simulink model "linearMSBR"  (R2016b)
settings: Solver=ode45  StartTime=0.0  StopTime=100.0  RelTol=1e-3
values from neighbouring files (symbols this model uses):
  A = zeros(16,16)    [simulinkmatrixconstructor.m]
  B = zeros(16,11)    [simulinkmatrixconstructor.m]
  mdotf_0 = (fPg1+fPg2+fPf1+fPf2+fPf3+fPf3)*P/cpf/(Tfhigh-Tflow)    (= 3034.32428551)    [simulinkmatrixconstructor.m]
  mfuelloop = 25*rhof*(1.32+1.22)    (= 8064.5)    [simulinkmatrixconstructor.m]
libraries: simulink x1
settings Model: Creator=gavin  LastModifiedBy=gavin

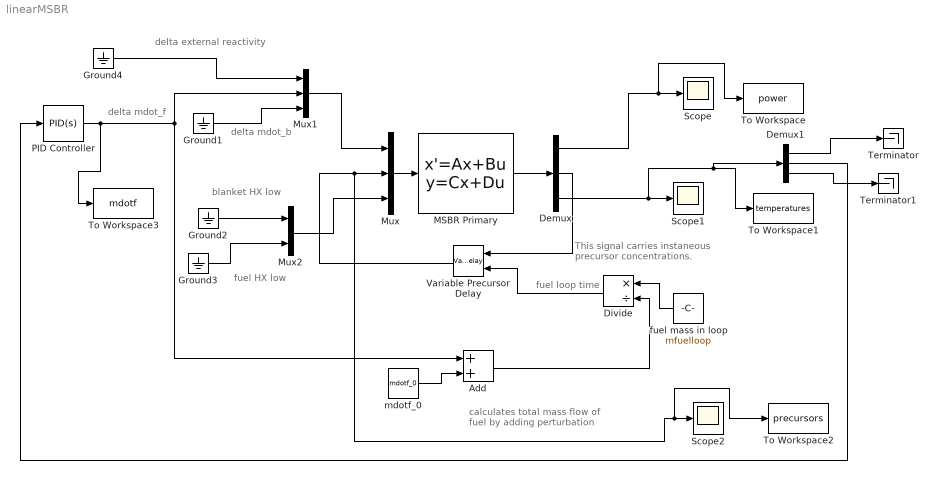
== system linearMSBR ==
  note: fuel HX low
  note: blanket HX low
  note: fuel loop time
  note: calculates total mass flow
      | of fuel by adding perturbation
  note: delta mdot_b
  note: delta mdot_f
  note: delta external reactivity
  note: This signal carries instaneous
      |  precursor concentrations.
  Add : Sum
  Demux : Demux  Outputs=[1 6 9]
  Demux1 : Demux  Outputs=[5 1 3]
  Divide : Product  Inputs=*/
  Ground{1..4} (4 alike) : Ground
  MSBR Primary : StateSpace  A=A  B=B  C=eye(16,16)  D=zeros(16,11)  X0=0  ContinuousStateAttributes='MSBR.state.variables'
  Mux : Mux  Inputs=[3 6 2]
  Mux1 : Mux  Inputs=3
  Mux2 : Mux  Inputs=2
  PID Controller : simulink/Continuous/PID Controller  Controller=PID  TimeDomain=Continuous-time  SampleTime=-1  IntegratorMethod=Forward Euler  FilterMethod=Forward Euler  Form=Parallel  UseFilter=on  ControllerParametersSource=internal  P=200  I=40  D=10  N=0.012270941775282  InitialConditionSource=internal  InitialConditionForIntegrator=0  InitialConditionForFilter=0  ExternalReset=none  LimitOutput=off  UpperSaturationLimit=inf  LowerSaturationLimit=-inf  LinearizeAsGain=on  AntiWindupMode=none  Kb=1  TrackingMode=off  Kt=1  PParamMin=[]  PParamMax=[]  IParamMin=[]  IParamMax=[]  DParamMin=[]  DParamMax=[]  NParamMin=[]  NParamMax=[]  KbParamMin=[]  KbParamMax=[]  KtParamMin=[]  KtParamMax=[]  POutMin=[]  POutMax=[]  IOutMin=[]  IOutMax=[]  DOutMin=[]  DOutMax=[]  NOutMin=[]  NOutMax=[]  KbOutMin=[]  KbOutMax=[]  KtOutMin=[]  KtOutMax=[]  IntegratorOutMin=[]  IntegratorOutMax=[]  FilterOutMin=[]  FilterOutMax=[]  SumOutMin=[]  SumOutMax=[]  SumI1OutMin=[]  SumI1OutMax=[]  SumI2OutMin=[]  SumI2OutMax=[]  SumI3OutMin=[]  SumI3OutMax=[]  SumDOutMin=[]  SumDOutMax=[]  SaturationOutMin=[]  SaturationOutMax=[]  IntegratorContinuousStateAttributes=''  IntegratorStateMustResolveToSignalObject=off  IntegratorRTWStateStorageClass=Auto  FilterContinuousStateAttributes=''  FilterStateMustResolveToSignalObject=off  FilterRTWStateStorageClass=Auto  DifferentiatorICPrevScaledInput=0  DifferentiatorOutMin=[]  DifferentiatorOutMax=[]
  Scope : Scope
  Scope1 : Scope
  Scope2 : Scope
  Terminator : Terminator
  Terminator1 : Terminator
  To Workspace : ToWorkspace  VariableName=power  SaveFormat=Timeseries  SampleTime=-1
  To Workspace1 : ToWorkspace  VariableName=temperatures  SaveFormat=Timeseries  SampleTime=-1
  To Workspace2 : ToWorkspace  VariableName=precursors  SaveFormat=Timeseries  SampleTime=-1
  To Workspace3 : ToWorkspace  VariableName=mdotf  SaveFormat=Timeseries  SampleTime=-1
  Variable Precursor Delay : VariableTransportDelay  MaximumDelay=10
  fuel mass in loop : Constant  Value=mfuelloop
  mdotf_0 : Constant  Value=mdotf_0
  wires:
  Mux/1 -> MSBR Primary/1
  MSBR Primary/1 -> Demux/1
  Demux/2 -> Variable Precursor Delay/1
  Demux/1 -> To Workspace/1, Scope/1
  Mux1/1 -> Mux/1
  PID Controller/1 -> To Workspace3/1, Mux1/2, Add/1
  Ground1/1 -> Mux1/3
  Mux2/1 -> Mux/3
  Ground2/1 -> Mux2/1
  Divide/1 -> Variable Precursor Delay/2
  fuel mass in loop/1 -> Divide/1
  mdotf_0/1 -> Add/2
  Add/1 -> Divide/2
  Demux/3 -> Demux1/1, To Workspace1/1, Scope1/1
  Variable Precursor Delay/1 -> To Workspace2/1, Scope2/1, Mux/2
  Ground4/1 -> Mux1/1
  Ground3/1 -> Mux2/2
  Demux1/1 -> Terminator/1
  Demux1/3 -> Terminator1/1
  Demux1/2 -> PID Controller/1
